simulink model "QR_Unitree_with_spine"  (R2021b)
settings: Solver=ode23t  StartTime=0.0  StopTime=10  FixedStep=1e-2  MaxStep=0.01  RelTol=1e-3  AbsTol=1e-3  EnableMultiTasking=on
values from neighbouring files (symbols this model uses):
  body_dim = [0.267 0.194 0.114]    [last_scores.mat]    (also in robotParameters.m)
  body_mass = 6.0    (= 6)    [CostOfTransport.m]    (also in last_scores.mat; robotParameters.m)
  delta_gait_front = 48    [PD_optimizedData_16Mar22_1632.mat]    (also in PD_optimizedData_16Mar22_2228_good.mat = 58; PD_optimizedData_17Mar22_1432_vel_walk_03735.mat = 56; PD_optimizedData_18Mar22_1518_right_direction.mat = 46; PD_optimizedData_18Mar22_1539.mat = 88)
  delta_gait_rear = 56    [PD_optimizedData_16Mar22_1632.mat]    (also in PD_optimizedData_16Mar22_2228_good.mat = 40; PD_optimizedData_17Mar22_1432_vel_walk_03735.mat = 6; PD_optimizedData_18Mar22_1518_right_direction.mat = 76; PD_optimizedData_18Mar22_1539.mat = 42)
  fem_der_front = [0 1.0471975512 -3.66519142919 -6.45771823238 -0.523598775598 5.41052068118 0]    [last_scores.mat]
  fem_der_rear = [0 -2.61799387799 -0.872664625997 1.2217304764 4.88692190558 1.3962634016 0]    [last_scores.mat]
  fem_motionFront = femur_motionFront    [CostFcnPDcontroll.m]    (also in CostFuncOptimizeSpine.m; last_scores.mat = [-2.12930168743 -2.33874119767 -2.26892802759 -2.12930168743; nonlinearContraints.m = deg2rad([x(1:N), x(1)]); nonlinearContraintsSpine.m = deg2rad([x(1:N), x(1)]))
  fem_motionRear = femur_motionRear    [CostFcnPDcontroll.m]    (also in CostFuncOptimizeSpine.m; last_scores.mat = [-2.09439510239 -2.12930168743 -2.16420827247 -2.19911485751; nonlinearContraints.m = deg2rad([x(2*N+1:3*N), x(2*N+1)]); nonlinearContraintsSpine.m = deg2rad([x(2*N+1:3*N), x(2*N+1)]))
  femur_height = 0.034    [last_scores.mat]    (also in robotParameters.m)
  femur_width = 0.0245    [last_scores.mat]    (also in robotParameters.m)
  gait_period = 1.2    [PD_optimizedData_16Mar22_1632.mat]    (also in PD_optimizedData_16Mar22_2228_good.mat; PD_optimizedData_17Mar22_1432_vel_walk_03735.mat; PD_optimizedData_18Mar22_1518_right_direction.mat; PD_optimizedData_18Mar22_1539.mat)
  ground = [20 2 0.1]    [last_scores.mat]    (also in robotParameters.m = [20 1.5 0.05])
  hip_mass = 0.595    [CostOfTransport.m]    (also in last_scores.mat; robotParameters.m)
  hip_radius = 0.046    [last_scores.mat]    (also in robotParameters.m)
  init_angs_F_front = deg2rad([-140 95])    [CostFcnPDcontroll.m]    (also in CostFuncOptimizeSpine.m = [q(1,1) q(2,1)]; last_scores.mat = [-2.12930168743 1.0471975512])
  init_angs_F_rear = deg2rad([-140 95])    [CostFcnPDcontroll.m]    (also in CostFuncOptimizeSpine.m = [q(1,1) q(2,1)]; last_scores.mat = [-2.09439510239 0.942477796077])
  init_angs_S_front = deg2rad([-140 95])    [CostFcnPDcontroll.m]    (also in CostFuncOptimizeSpine.m = [q(1,2) q(2,2)]; last_scores.mat = [-2.20972645936 0.894446335062])
  init_angs_S_rear = deg2rad([-140 95])    [CostFcnPDcontroll.m]    (also in CostFuncOptimizeSpine.m = [q(1,2) q(2,2)]; last_scores.mat = [-2.20954326961 0.961688146461])
  max_torque = 33.5    [last_scores.mat]    (also in robotParameters.m)
  N = (numel(x)-2)/4    [nonlinearContraints.m]    (also in nonlinearContraintsSpine.m = (numel(x)-5)/4; pampam.m = numel(params)/2)
  tib_der_front = [0 -1.74532925199 0.349065850399 0 1.57079632679 1.74532925199 0]    [last_scores.mat]
  tib_der_rear = [0 0.698131700798 -1.3962634016 3.31612557879 2.44346095279 -4.01425727959 0]    [last_scores.mat]
  tib_motionFront = tibia_motionFront    [CostFcnPDcontroll.m]    (also in CostFuncOptimizeSpine.m; last_scores.mat = [1.0471975512 0.977384381117 0.872664625997 0.977384381117 1; nonlinearContraints.m = deg2rad([x(N+1:2*N), x(N+1)]); nonlinearContraintsSpine.m = deg2rad([x(N+1:2*N), x(N+1)]))
  tib_motionRear = tibia_motionRear    [CostFcnPDcontroll.m]    (also in CostFuncOptimizeSpine.m; last_scores.mat = [0.942477796077 1.08210413624 0.733038285838 1.18682389136 1; nonlinearContraints.m = deg2rad([x(3*N+1:4*N), x(3*N+1)]); nonlinearContraintsSpine.m = deg2rad([x(3*N+1:4*N), x(3*N+1)]))
  tibia_height = 0.016    [last_scores.mat]    (also in robotParameters.m)
  tibia_width = 0.016    [last_scores.mat]    (also in robotParameters.m)
  traj_times = [0 0.2 0.4 0.6 0.8 1 1.2]    [PD_optimizedData_16Mar22_1632.mat]    (also in PD_optimizedData_16Mar22_2228_good.mat; PD_optimizedData_17Mar22_1432_vel_walk_03735.mat; PD_optimizedData_18Mar22_1518_right_direction.mat; PD_optimizedData_18Mar22_1539.mat)
  tsTraj = 0.01    [last_scores.mat]    (also in pampam.m; robotParameters.m)
undefined symbols (not defined in the file or in its folder): X, Y, Z
libraries: sm_lib x39, nesl_utility x7, robotcorelib x4, QR_library x4, simulink x4
(part 2 of 2)

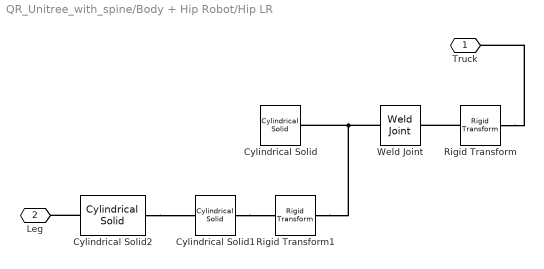
== system QR_Unitree_with_spine/Body + Hip Robot/Hip LR ==
  Cylindrical Solid : sm_lib/Body Elements/Cylindrical Solid  GraphicAmbientColor=[0.15 0.15 0.15 1.0]  BasedOnType=Density  CenterOfMass=[0 0 0]  CenterOfMassUnits=m  GraphicDiffuseColor=[0.0 0.2 0.6]  CylinderLength=hip_length  CylinderLengthUnits=m  CylinderRadius=hip_radius  CylinderRadiusUnits=m  Density=1000  DensityUnits=kg/m^3  DoExposeReferenceFrame=on  GraphicEmissiveColor=[0.0 0.0 0.0 1.0]  ExportEntireGeometry=off  SerializedFrames=<Frames/>  MarkerShape=Sphere  MarkerSize=10  GraphicType=FromGeometry  InertiaType=PointMass  Mass=hip_mass/2  MassUnits=kg  MomentsOfInertia=[1 1 1]  MomentsOfInertiaUnits=kg*m^2  GraphicOpacity=1.0  ProductsOfInertia=[0 0 0]  ProductsOfInertiaUnits=kg*m^2  GraphicShininess=75  GraphicSpecularColor=[0.5 0.5 0.5 1.0]  GraphicVisPropType=SimpleVisualProperties
  Cylindrical Solid1 : sm_lib/Body Elements/Cylindrical Solid  GraphicAmbientColor=[0.15 0.15 0.15 1.0]  BasedOnType=Density  CenterOfMass=[0 0 0]  CenterOfMassUnits=m  GraphicDiffuseColor=[0.2 0.0 0.8]  CylinderLength=hip_length  CylinderLengthUnits=m  CylinderRadius=hip_radius  CylinderRadiusUnits=m  Density=1000  DensityUnits=kg/m^3  DoExposeReferenceFrame=on  GraphicEmissiveColor=[0.0 0.0 0.0 1.0]  ExportEntireGeometry=off  SerializedFrames=<Frames><Frame><Id>Frame1</Id><Value><Name>Leg</Name><Origin><Source>GeometricFeature</Source><FeatureName>bottom surface</FeatureName></Origin><PrimaryAxis><DefinedDirection>+Z</DefinedDirection><Source>ReferenceFrame</Source><SourceDirection>+Z</SourceDirection><FeatureName></FeatureName></PrimaryAxis><SecondaryAxis><DefinedDirection>+X</DefinedDirection><Source>ReferenceFrame</Source><SourceDirection>+X</SourceDirection><FeatureName></FeatureName></SecondaryAxis></Value></Frame></Frames>  MarkerShape=Sphere  MarkerSize=10  GraphicType=FromGeometry  InertiaType=PointMass  Mass=hip_mass/2  MassUnits=kg  MomentsOfInertia=[1 1 1]  MomentsOfInertiaUnits=kg*m^2  GraphicOpacity=1.0  ProductsOfInertia=[0 0 0]  ProductsOfInertiaUnits=kg*m^2  GraphicShininess=75  GraphicSpecularColor=[0.5 0.5 0.5 1.0]  GraphicVisPropType=SimpleVisualProperties
  Cylindrical Solid2 : sm_lib/Body Elements/Cylindrical Solid  GraphicAmbientColor=[0.15 0.15 0.15 1.0]  BasedOnType=Density  CenterOfMass=[0 0 0]  CenterOfMassUnits=m  GraphicDiffuseColor=[0.2 0.2 1.0]  CylinderLength=femur_width  CylinderLengthUnits=m  CylinderRadius=hip_radius-0.01  CylinderRadiusUnits=m  Density=1000  DensityUnits=kg/m^3  DoExposeReferenceFrame=on  GraphicEmissiveColor=[0.0 0.0 0.0 1.0]  ExportEntireGeometry=off  SerializedFrames=<Frames><Frame><Id>Frame1</Id><Value><Name>hip_joint</Name><Origin><Source>GeometricFeature</Source><FeatureName>top surface</FeatureName></Origin><PrimaryAxis><DefinedDirection>+Z</DefinedDirection><Source>ReferenceFrame</Source><SourceDirection>+Z</SourceDirection><FeatureName></FeatureName></PrimaryAxis><SecondaryAxis><DefinedDirection>+X</DefinedDirection><Source>ReferenceFrame</Source><SourceDirection>+X</SourceDirection><FeatureName></FeatureName></SecondaryAxis></Value></Frame></Frames>  MarkerShape=Sphere  MarkerSize=10  GraphicType=FromGeometry  InertiaType=CalculateFromGeometry  Mass=1  MassUnits=kg  MomentsOfInertia=[1 1 1]  MomentsOfInertiaUnits=kg*m^2  GraphicOpacity=1.0  ProductsOfInertia=[0 0 0]  ProductsOfInertiaUnits=kg*m^2  GraphicShininess=75  GraphicSpecularColor=[0.5 0.5 0.5 1.0]  GraphicVisPropType=SimpleVisualProperties
  Rigid Transform : sm_lib/Frames and Transforms/Rigid Transform  TranslationMethod=Cartesian  TranslationStandardOffset=0  TranslationLengthUnit=m  TranslationStandardAxis=+Z  TranslationCartesianOffset=offset_LR  TranslationROffset=0  TranslationROffsetUnits=m  TranslationZOffset=0  TranslationZOffsetUnits=m  TranslationThetaOffset=0  TranslationThetaOffsetUnits=deg  RotationMethod=StandardAxis  RotationAngleUnits=rad  RotationStandardAxis=+X  RotationAngle=pi/2  RotationArbitraryAxis=[0 0 1]  FollAlignAxisA=+X  BaseAlignAxisA=+Y  FollAlignAxisB=+Y  BaseAlignAxisB=+Z  RotationSequenceAxes=FollowerAxes  RotationSequence=XYX  RotationSequenceAngles=[0 0 0]  RotationSequenceAnglesUnits=deg  RotationMatrix=[1 0 0; 0 1 0; 0 0 1]
  Rigid Transform1 : sm_lib/Frames and Transforms/Rigid Transform  TranslationMethod=StandardAxis  TranslationStandardOffset=hip_offset  TranslationLengthUnit=m  TranslationStandardAxis=-Z  TranslationCartesianOffset=[0 0 0]  TranslationROffset=0  TranslationROffsetUnits=m  TranslationZOffset=0  TranslationZOffsetUnits=m  TranslationThetaOffset=0  TranslationThetaOffsetUnits=deg  RotationMethod=None  RotationAngleUnits=rad  RotationStandardAxis=+X  RotationAngle=pi/2  RotationArbitraryAxis=[0 0 1]  FollAlignAxisA=+X  BaseAlignAxisA=+Y  FollAlignAxisB=+Y  BaseAlignAxisB=+Z  RotationSequenceAxes=FollowerAxes  RotationSequence=XYX  RotationSequenceAngles=[0 0 0]  RotationSequenceAnglesUnits=deg  RotationMatrix=[1 0 0; 0 1 0; 0 0 1]
  Weld Joint : sm_lib/Joints/Weld Joint  JointMode=Normal  SenseConstraintForce=off  SenseConstraintForceX=off  SenseConstraintForceY=off  SenseConstraintForceZ=off  SenseConstraintTorque=off  SenseConstraintTorqueX=off  SenseConstraintTorqueY=off  SenseConstraintTorqueZ=off  SenseTotalForce=off  SenseTotalForceX=off  SenseTotalForceY=off  SenseTotalForceZ=off  SenseTotalTorque=off  SenseTotalTorqueX=off  SenseTotalTorqueY=off  SenseTotalTorqueZ=off  CompositeWrenchDir=FollowerOnBase  CompositeWrenchFrame=BaseFrame
  Truck : PMIOPort  Side=Left
  Leg : PMIOPort  Port=2  Side=Right
  connections:
  Cylindrical Solid1/RConn1 -- Rigid Transform1/RConn1
  Cylindrical Solid2/RConn1 -- Leg/RConn1
  Rigid Transform/LConn1 -- Truck/RConn1
  Rigid Transform/RConn1 -- Weld Joint/LConn1
  Rigid Transform1/LConn1 -- Cylindrical Solid/RConn1 -- Weld Joint/RConn1
  Cylindrical Solid2/LConn1 -- Cylindrical Solid1/LConn1

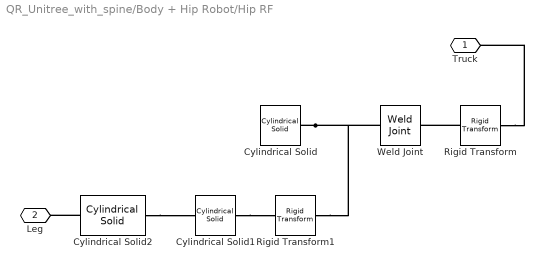
== system QR_Unitree_with_spine/Body + Hip Robot/Hip RF ==
  Cylindrical Solid : sm_lib/Body Elements/Cylindrical Solid  GraphicAmbientColor=[0.15 0.15 0.15 1.0]  BasedOnType=Density  CenterOfMass=[0 0 0]  CenterOfMassUnits=m  GraphicDiffuseColor=[0.0 0.2 0.6]  CylinderLength=hip_length  CylinderLengthUnits=m  CylinderRadius=hip_radius  CylinderRadiusUnits=m  Density=1000  DensityUnits=kg/m^3  DoExposeReferenceFrame=on  GraphicEmissiveColor=[0.0 0.0 0.0 1.0]  ExportEntireGeometry=off  SerializedFrames=<Frames/>  MarkerShape=Sphere  MarkerSize=10  GraphicType=FromGeometry  InertiaType=PointMass  Mass=hip_mass/2  MassUnits=kg  MomentsOfInertia=[1 1 1]  MomentsOfInertiaUnits=kg*m^2  GraphicOpacity=1.0  ProductsOfInertia=[0 0 0]  ProductsOfInertiaUnits=kg*m^2  GraphicShininess=75  GraphicSpecularColor=[0.5 0.5 0.5 1.0]  GraphicVisPropType=SimpleVisualProperties
  Cylindrical Solid1 : sm_lib/Body Elements/Cylindrical Solid  GraphicAmbientColor=[0.15 0.15 0.15 1.0]  BasedOnType=Density  CenterOfMass=[0 0 0]  CenterOfMassUnits=m  GraphicDiffuseColor=[0.2 0.0 0.8]  CylinderLength=hip_length  CylinderLengthUnits=m  CylinderRadius=hip_radius  CylinderRadiusUnits=m  Density=1000  DensityUnits=kg/m^3  DoExposeReferenceFrame=on  GraphicEmissiveColor=[0.0 0.0 0.0 1.0]  ExportEntireGeometry=off  SerializedFrames=<Frames><Frame><Id>Frame1</Id><Value><Name>Leg</Name><Origin><Source>GeometricFeature</Source><FeatureName>top surface</FeatureName></Origin><PrimaryAxis><DefinedDirection>+Z</DefinedDirection><Source>ReferenceFrame</Source><SourceDirection>+Z</SourceDirection><FeatureName></FeatureName></PrimaryAxis><SecondaryAxis><DefinedDirection>+X</DefinedDirection><Source>ReferenceFrame</Source><SourceDirection>+X</SourceDirection><FeatureName></FeatureName></SecondaryAxis></Value></Frame></Frames>  MarkerShape=Sphere  MarkerSize=10  GraphicType=FromGeometry  InertiaType=PointMass  Mass=hip_mass/2  MassUnits=kg  MomentsOfInertia=[1 1 1]  MomentsOfInertiaUnits=kg*m^2  GraphicOpacity=1.0  ProductsOfInertia=[0 0 0]  ProductsOfInertiaUnits=kg*m^2  GraphicShininess=75  GraphicSpecularColor=[0.5 0.5 0.5 1.0]  GraphicVisPropType=SimpleVisualProperties
  Cylindrical Solid2 : sm_lib/Body Elements/Cylindrical Solid  GraphicAmbientColor=[0.15 0.15 0.15 1.0]  BasedOnType=Density  CenterOfMass=[0 0 0]  CenterOfMassUnits=m  GraphicDiffuseColor=[0.2 0.2 1.0]  CylinderLength=femur_width  CylinderLengthUnits=m  CylinderRadius=hip_radius-0.01  CylinderRadiusUnits=m  Density=1000  DensityUnits=kg/m^3  DoExposeReferenceFrame=on  GraphicEmissiveColor=[0.0 0.0 0.0 1.0]  ExportEntireGeometry=off  SerializedFrames=<Frames><Frame><Id>Frame1</Id><Value><Name>hip_joint</Name><Origin><Source>GeometricFeature</Source><FeatureName>bottom surface</FeatureName></Origin><PrimaryAxis><DefinedDirection>+Z</DefinedDirection><Source>ReferenceFrame</Source><SourceDirection>+Z</SourceDirection><FeatureName></FeatureName></PrimaryAxis><SecondaryAxis><DefinedDirection>+X</DefinedDirection><Source>ReferenceFrame</Source><SourceDirection>+X</SourceDirection><FeatureName></FeatureName></SecondaryAxis></Value></Frame></Frames>  MarkerShape=Sphere  MarkerSize=10  GraphicType=FromGeometry  InertiaType=CalculateFromGeometry  Mass=1  MassUnits=kg  MomentsOfInertia=[1 1 1]  MomentsOfInertiaUnits=kg*m^2  GraphicOpacity=1.0  ProductsOfInertia=[0 0 0]  ProductsOfInertiaUnits=kg*m^2  GraphicShininess=75  GraphicSpecularColor=[0.5 0.5 0.5 1.0]  GraphicVisPropType=SimpleVisualProperties
  Rigid Transform : sm_lib/Frames and Transforms/Rigid Transform  TranslationMethod=Cartesian  TranslationStandardOffset=0  TranslationLengthUnit=m  TranslationStandardAxis=+Z  TranslationCartesianOffset=offset_RF  TranslationROffset=0  TranslationROffsetUnits=m  TranslationZOffset=0  TranslationZOffsetUnits=m  TranslationThetaOffset=0  TranslationThetaOffsetUnits=deg  RotationMethod=StandardAxis  RotationAngleUnits=rad  RotationStandardAxis=+X  RotationAngle=pi/2  RotationArbitraryAxis=[0 0 1]  FollAlignAxisA=+X  BaseAlignAxisA=+Y  FollAlignAxisB=+Y  BaseAlignAxisB=+Z  RotationSequenceAxes=FollowerAxes  RotationSequence=XYX  RotationSequenceAngles=[0 0 0]  RotationSequenceAnglesUnits=deg  RotationMatrix=[1 0 0; 0 1 0; 0 0 1]
  Rigid Transform1 : sm_lib/Frames and Transforms/Rigid Transform  TranslationMethod=StandardAxis  TranslationStandardOffset=hip_offset  TranslationLengthUnit=m  TranslationStandardAxis=+Z  TranslationCartesianOffset=[0 0 0]  TranslationROffset=0  TranslationROffsetUnits=m  TranslationZOffset=0  TranslationZOffsetUnits=m  TranslationThetaOffset=0  TranslationThetaOffsetUnits=deg  RotationMethod=None  RotationAngleUnits=rad  RotationStandardAxis=+X  RotationAngle=pi/2  RotationArbitraryAxis=[0 0 1]  FollAlignAxisA=+X  BaseAlignAxisA=+Y  FollAlignAxisB=+Y  BaseAlignAxisB=+Z  RotationSequenceAxes=FollowerAxes  RotationSequence=XYX  RotationSequenceAngles=[0 0 0]  RotationSequenceAnglesUnits=deg  RotationMatrix=[1 0 0; 0 1 0; 0 0 1]
  Weld Joint : sm_lib/Joints/Weld Joint  JointMode=Normal  SenseConstraintForce=off  SenseConstraintForceX=off  SenseConstraintForceY=off  SenseConstraintForceZ=off  SenseConstraintTorque=off  SenseConstraintTorqueX=off  SenseConstraintTorqueY=off  SenseConstraintTorqueZ=off  SenseTotalForce=off  SenseTotalForceX=off  SenseTotalForceY=off  SenseTotalForceZ=off  SenseTotalTorque=off  SenseTotalTorqueX=off  SenseTotalTorqueY=off  SenseTotalTorqueZ=off  CompositeWrenchDir=FollowerOnBase  CompositeWrenchFrame=BaseFrame
  Truck : PMIOPort  Side=Left
  Leg : PMIOPort  Port=2  Side=Right
  connections:
  Cylindrical Solid1/RConn1 -- Rigid Transform1/RConn1
  Cylindrical Solid2/RConn1 -- Leg/RConn1
  Rigid Transform/LConn1 -- Truck/RConn1
  Rigid Transform/RConn1 -- Weld Joint/LConn1
  Cylindrical Solid/RConn1 -- Weld Joint/RConn1 -- Rigid Transform1/LConn1
  Cylindrical Solid2/LConn1 -- Cylindrical Solid1/LConn1

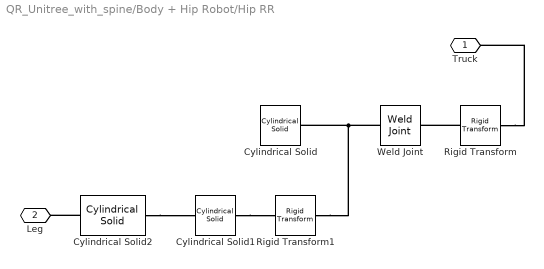
== system QR_Unitree_with_spine/Body + Hip Robot/Hip RR ==
  Cylindrical Solid : sm_lib/Body Elements/Cylindrical Solid  GraphicAmbientColor=[0.15 0.15 0.15 1.0]  BasedOnType=Density  CenterOfMass=[0 0 0]  CenterOfMassUnits=m  GraphicDiffuseColor=[0.0 0.2 0.6]  CylinderLength=hip_length  CylinderLengthUnits=m  CylinderRadius=hip_radius  CylinderRadiusUnits=m  Density=1000  DensityUnits=kg/m^3  DoExposeReferenceFrame=on  GraphicEmissiveColor=[0.0 0.0 0.0 1.0]  ExportEntireGeometry=off  SerializedFrames=<Frames/>  MarkerShape=Sphere  MarkerSize=10  GraphicType=FromGeometry  InertiaType=PointMass  Mass=hip_mass/2  MassUnits=kg  MomentsOfInertia=[1 1 1]  MomentsOfInertiaUnits=kg*m^2  GraphicOpacity=1.0  ProductsOfInertia=[0 0 0]  ProductsOfInertiaUnits=kg*m^2  GraphicShininess=75  GraphicSpecularColor=[0.5 0.5 0.5 1.0]  GraphicVisPropType=SimpleVisualProperties
  Cylindrical Solid1 : sm_lib/Body Elements/Cylindrical Solid  GraphicAmbientColor=[0.15 0.15 0.15 1.0]  BasedOnType=Density  CenterOfMass=[0 0 0]  CenterOfMassUnits=m  GraphicDiffuseColor=[0.2 0.0 0.8]  CylinderLength=hip_length  CylinderLengthUnits=m  CylinderRadius=hip_radius  CylinderRadiusUnits=m  Density=1000  DensityUnits=kg/m^3  DoExposeReferenceFrame=on  GraphicEmissiveColor=[0.0 0.0 0.0 1.0]  ExportEntireGeometry=off  SerializedFrames=<Frames><Frame><Id>Frame1</Id><Value><Name>Leg</Name><Origin><Source>GeometricFeature</Source><FeatureName>top surface</FeatureName></Origin><PrimaryAxis><DefinedDirection>+Z</DefinedDirection><Source>ReferenceFrame</Source><SourceDirection>+Z</SourceDirection><FeatureName></FeatureName></PrimaryAxis><SecondaryAxis><DefinedDirection>+X</DefinedDirection><Source>ReferenceFrame</Source><SourceDirection>+X</SourceDirection><FeatureName></FeatureName></SecondaryAxis></Value></Frame></Frames>  MarkerShape=Sphere  MarkerSize=10  GraphicType=FromGeometry  InertiaType=PointMass  Mass=hip_mass/2  MassUnits=kg  MomentsOfInertia=[1 1 1]  MomentsOfInertiaUnits=kg*m^2  GraphicOpacity=1.0  ProductsOfInertia=[0 0 0]  ProductsOfInertiaUnits=kg*m^2  GraphicShininess=75  GraphicSpecularColor=[0.5 0.5 0.5 1.0]  GraphicVisPropType=SimpleVisualProperties
  Cylindrical Solid2 : sm_lib/Body Elements/Cylindrical Solid  GraphicAmbientColor=[0.15 0.15 0.15 1.0]  BasedOnType=Density  CenterOfMass=[0 0 0]  CenterOfMassUnits=m  GraphicDiffuseColor=[0.2 0.2 1.0]  CylinderLength=femur_width  CylinderLengthUnits=m  CylinderRadius=hip_radius-0.01  CylinderRadiusUnits=m  Density=1000  DensityUnits=kg/m^3  DoExposeReferenceFrame=on  GraphicEmissiveColor=[0.0 0.0 0.0 1.0]  ExportEntireGeometry=off  SerializedFrames=<Frames><Frame><Id>Frame1</Id><Value><Name>hip_joint</Name><Origin><Source>GeometricFeature</Source><FeatureName>bottom surface</FeatureName></Origin><PrimaryAxis><DefinedDirection>+Z</DefinedDirection><Source>ReferenceFrame</Source><SourceDirection>+Z</SourceDirection><FeatureName></FeatureName></PrimaryAxis><SecondaryAxis><DefinedDirection>+X</DefinedDirection><Source>ReferenceFrame</Source><SourceDirection>+X</SourceDirection><FeatureName></FeatureName></SecondaryAxis></Value></Frame></Frames>  MarkerShape=Sphere  MarkerSize=10  GraphicType=FromGeometry  InertiaType=CalculateFromGeometry  Mass=1  MassUnits=kg  MomentsOfInertia=[1 1 1]  MomentsOfInertiaUnits=kg*m^2  GraphicOpacity=1.0  ProductsOfInertia=[0 0 0]  ProductsOfInertiaUnits=kg*m^2  GraphicShininess=75  GraphicSpecularColor=[0.5 0.5 0.5 1.0]  GraphicVisPropType=SimpleVisualProperties
  Rigid Transform : sm_lib/Frames and Transforms/Rigid Transform  TranslationMethod=Cartesian  TranslationStandardOffset=0  TranslationLengthUnit=m  TranslationStandardAxis=+Z  TranslationCartesianOffset=offset_RR  TranslationROffset=0  TranslationROffsetUnits=m  TranslationZOffset=0  TranslationZOffsetUnits=m  TranslationThetaOffset=0  TranslationThetaOffsetUnits=deg  RotationMethod=StandardAxis  RotationAngleUnits=rad  RotationStandardAxis=+X  RotationAngle=pi/2  RotationArbitraryAxis=[0 0 1]  FollAlignAxisA=+X  BaseAlignAxisA=+Y  FollAlignAxisB=+Y  BaseAlignAxisB=+Z  RotationSequenceAxes=FollowerAxes  RotationSequence=XYX  RotationSequenceAngles=[0 0 0]  RotationSequenceAnglesUnits=deg  RotationMatrix=[1 0 0; 0 1 0; 0 0 1]
  Rigid Transform1 : sm_lib/Frames and Transforms/Rigid Transform  TranslationMethod=StandardAxis  TranslationStandardOffset=hip_offset  TranslationLengthUnit=m  TranslationStandardAxis=+Z  TranslationCartesianOffset=[0 0 0]  TranslationROffset=0  TranslationROffsetUnits=m  TranslationZOffset=0  TranslationZOffsetUnits=m  TranslationThetaOffset=0  TranslationThetaOffsetUnits=deg  RotationMethod=None  RotationAngleUnits=rad  RotationStandardAxis=+X  RotationAngle=pi/2  RotationArbitraryAxis=[0 0 1]  FollAlignAxisA=+X  BaseAlignAxisA=+Y  FollAlignAxisB=+Y  BaseAlignAxisB=+Z  RotationSequenceAxes=FollowerAxes  RotationSequence=XYX  RotationSequenceAngles=[0 0 0]  RotationSequenceAnglesUnits=deg  RotationMatrix=[1 0 0; 0 1 0; 0 0 1]
  Weld Joint : sm_lib/Joints/Weld Joint  JointMode=Normal  SenseConstraintForce=off  SenseConstraintForceX=off  SenseConstraintForceY=off  SenseConstraintForceZ=off  SenseConstraintTorque=off  SenseConstraintTorqueX=off  SenseConstraintTorqueY=off  SenseConstraintTorqueZ=off  SenseTotalForce=off  SenseTotalForceX=off  SenseTotalForceY=off  SenseTotalForceZ=off  SenseTotalTorque=off  SenseTotalTorqueX=off  SenseTotalTorqueY=off  SenseTotalTorqueZ=off  CompositeWrenchDir=FollowerOnBase  CompositeWrenchFrame=BaseFrame
  Truck : PMIOPort  Side=Left
  Leg : PMIOPort  Port=2  Side=Right
  connections:
  Cylindrical Solid2/LConn1 -- Cylindrical Solid1/LConn1
  Weld Joint/RConn1 -- Cylindrical Solid/RConn1 -- Rigid Transform1/LConn1
  Rigid Transform/RConn1 -- Weld Joint/LConn1
  Rigid Transform/LConn1 -- Truck/RConn1
  Cylindrical Solid2/RConn1 -- Leg/RConn1
  Cylindrical Solid1/RConn1 -- Rigid Transform1/RConn1

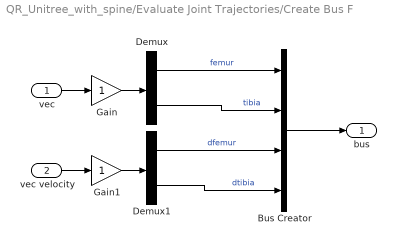
== system QR_Unitree_with_spine/Evaluate Joint Trajectories/Create Bus F ==
  vec : Inport
  vec velocity : Inport  Port=2
  Bus Creator : BusCreator  Inputs=4
  Demux : Demux  Outputs=2
  Demux1 : Demux  Outputs=2
  Gain : Gain
  Gain1 : Gain
  bus : Outport  VectorParamsAs1DForOutWhenUnconnected=off
  wires:
  Bus Creator/1 -> bus/1
  vec/1 -> Gain/1
  Demux/2 -> Bus Creator/2  "tibia"
  Demux/1 -> Bus Creator/1  "femur"
  Gain/1 -> Demux/1
  Gain1/1 -> Demux1/1
  Demux1/1 -> Bus Creator/3  "dfemur"
  Demux1/2 -> Bus Creator/4  "dtibia"
  vec velocity/1 -> Gain1/1

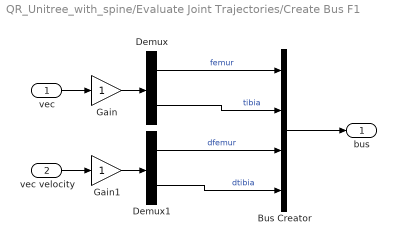
== system QR_Unitree_with_spine/Evaluate Joint Trajectories/Create Bus F1 ==
  vec : Inport
  vec velocity : Inport  Port=2
  Bus Creator : BusCreator  Inputs=4
  Demux : Demux  Outputs=2
  Demux1 : Demux  Outputs=2
  Gain : Gain
  Gain1 : Gain
  bus : Outport  VectorParamsAs1DForOutWhenUnconnected=off
  wires:
  vec velocity/1 -> Gain1/1
  Demux1/2 -> Bus Creator/4  "dtibia"
  Demux1/1 -> Bus Creator/3  "dfemur"
  Gain1/1 -> Demux1/1
  Gain/1 -> Demux/1
  Demux/1 -> Bus Creator/1  "femur"
  Demux/2 -> Bus Creator/2  "tibia"
  vec/1 -> Gain/1
  Bus Creator/1 -> bus/1

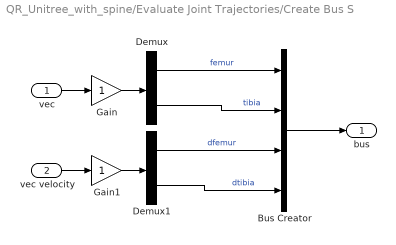
== system QR_Unitree_with_spine/Evaluate Joint Trajectories/Create Bus S ==
  vec : Inport
  vec velocity : Inport  Port=2
  Bus Creator : BusCreator  Inputs=4
  Demux : Demux  Outputs=2
  Demux1 : Demux  Outputs=2
  Gain : Gain
  Gain1 : Gain
  bus : Outport  VectorParamsAs1DForOutWhenUnconnected=off
  wires:
  vec velocity/1 -> Gain1/1
  Demux1/2 -> Bus Creator/4  "dtibia"
  Demux1/1 -> Bus Creator/3  "dfemur"
  Gain1/1 -> Demux1/1
  Gain/1 -> Demux/1
  Demux/1 -> Bus Creator/1  "femur"
  Demux/2 -> Bus Creator/2  "tibia"
  vec/1 -> Gain/1
  Bus Creator/1 -> bus/1

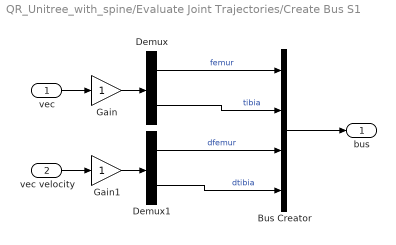
== system QR_Unitree_with_spine/Evaluate Joint Trajectories/Create Bus S1 ==
  vec : Inport
  vec velocity : Inport  Port=2
  Bus Creator : BusCreator  Inputs=4
  Demux : Demux  Outputs=2
  Demux1 : Demux  Outputs=2
  Gain : Gain
  Gain1 : Gain
  bus : Outport  VectorParamsAs1DForOutWhenUnconnected=off
  wires:
  Bus Creator/1 -> bus/1
  vec/1 -> Gain/1
  Demux/2 -> Bus Creator/2  "tibia"
  Demux/1 -> Bus Creator/1  "femur"
  Gain/1 -> Demux/1
  Gain1/1 -> Demux1/1
  Demux1/1 -> Bus Creator/3  "dfemur"
  Demux1/2 -> Bus Creator/4  "dtibia"
  vec velocity/1 -> Gain1/1
